simulink model "NavigationSystem"  (R2018b)
settings: Solver=ode4  StartTime=0.0  StopTime=2000  FixedStep=S_time  RelTol=1e-3
InitFcn:
  | run('DataInitial.m')
StopFcn:
  | run('PNPlot.m')
values from neighbouring files (symbols this model uses):
  GM = 3.986e5    (= 398600)    [DataInitial.m]
  N_PN = 5    [DataInitial.m]
  P0_M = [4510.1;4510.1]    [DataInitial.m]
  P0_T = [0;6378.2]    [DataInitial.m]
  V0_M = [2.0056;5.9535]    [DataInitial.m]
  V0_T = [6.7856;2.8801]    [DataInitial.m]
libraries: simulink x1
settings Model: Creator=Administrator  LastModifiedBy=Administrator

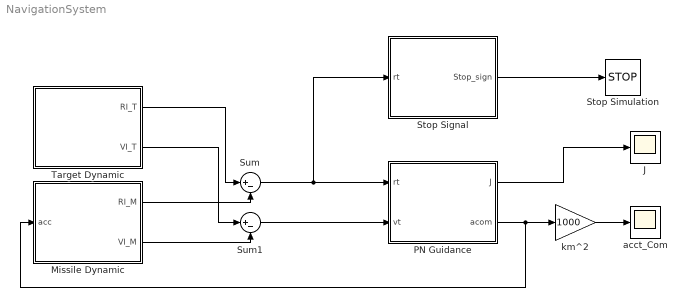
== system NavigationSystem ==
  J : Scope
  Missile Dynamic : Subsystem  mask(导弹设置){P0_M=P0_M, V0_M=V0_M}
      mask prompts: P0_M "导弹初始位置（km）"; V0_M "导弹初始速度（km/s)"
      mask help: 在这里设置导弹的初始位置和速度
  PN Guidance : Subsystem
  Stop Signal : Subsystem
  Stop Simulation : Stop
  Sum : Sum  Inputs=|+-
  Sum1 : Sum  Inputs=|+-
  Target Dynamic : Subsystem  mask(目标设置){P0_T=P0_T, V0_T=V0_T}
      mask prompts: P0_T "目标初始位置（km)"; V0_T "目标初始速度（km/s）"
      mask help: 在这里设置目标的初始位置和速度
  acct_Com : Scope
  km^2 : Gain  Gain=1000
  wires:
  Stop Signal/1(Stop_sign) -> Stop Simulation/1
  Target Dynamic/1(RI_T) -> Sum/1
  Target Dynamic/2(VI_T) -> Sum1/1
  Sum/1 -> Stop Signal/1(rt), PN Guidance/1(rt)
  Sum1/1 -> PN Guidance/2(vt)
  PN Guidance/1(J) -> J/1
  PN Guidance/2(acom) -> Missile Dynamic/1(acc), km^2/1
  km^2/1 -> acct_Com/1
  Missile Dynamic/1(RI_M) -> Sum/2
  Missile Dynamic/2(VI_M) -> Sum1/2

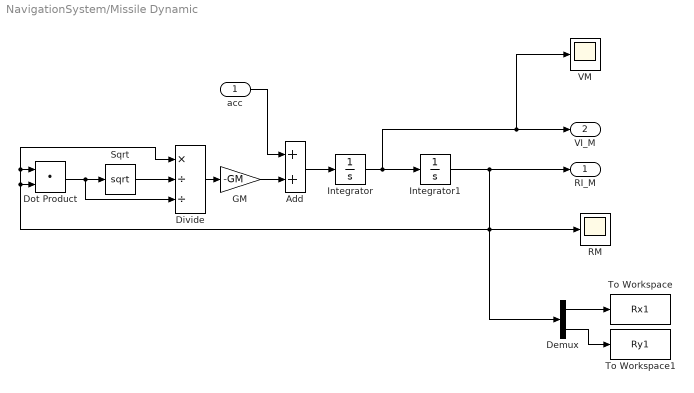
== system NavigationSystem/Missile Dynamic ==
  acc : Inport
  Add : Sum
  Demux : Demux  Outputs=2
  Divide : Product  Inputs=*//
  Dot Product : DotProduct  InputSameDT=on  OutDataTypeStr=Inherit: Inherit via internal rule
  GM : Gain  Gain=-GM
  Integrator : Integrator  InitialCondition=V0_M
  Integrator1 : Integrator  InitialCondition=P0_M
  RM : Scope
  Sqrt : Sqrt  SaturateOnIntegerOverflow=on
  To Workspace : ToWorkspace  VariableName=Rx1  SaveFormat=Timeseries  SampleTime=-1
  To Workspace1 : ToWorkspace  VariableName=Ry1  SaveFormat=Timeseries  SampleTime=-1
  VM : Scope
  RI_M : Outport
  VI_M : Outport  Port=2
  wires:
  Sqrt/1 -> Divide/2
  Integrator/1 -> VM/1, VI_M/1, Integrator1/1
  Dot Product/1 -> Divide/3, Sqrt/1
  Integrator1/1 -> Demux/1, Dot Product/1, Divide/1, Dot Product/2, RM/1, RI_M/1
  Divide/1 -> GM/1
  GM/1 -> Add/2
  Add/1 -> Integrator/1
  acc/1 -> Add/1
  Demux/1 -> To Workspace/1
  Demux/2 -> To Workspace1/1

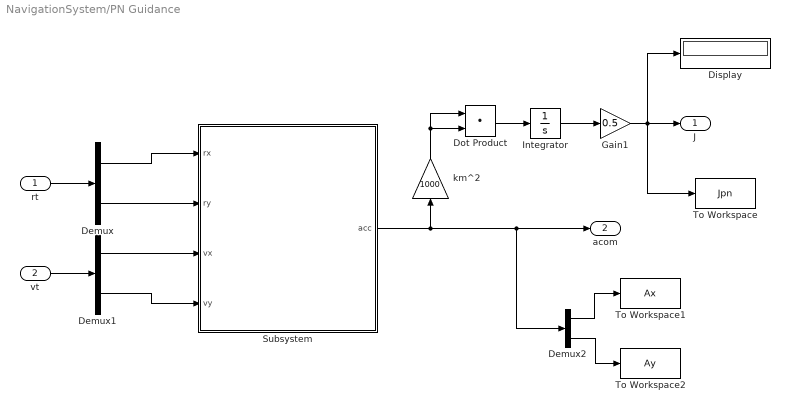
== system NavigationSystem/PN Guidance ==
  rt : Inport
  vt : Inport  Port=2
  Demux : Demux  Outputs=2
  Demux1 : Demux  Outputs=2
  Demux2 : Demux  Outputs=2
  Display : Display
  Dot Product : DotProduct  InputSameDT=on  OutDataTypeStr=Inherit: Inherit via internal rule
  Gain1 : Gain  Gain=0.5
  Integrator : Integrator
  Subsystem : Subsystem
  To Workspace : ToWorkspace  VariableName=Jpn  SaveFormat=Timeseries  SampleTime=-1
  To Workspace1 : ToWorkspace  VariableName=Ax  SaveFormat=Timeseries  SampleTime=-1
  To Workspace2 : ToWorkspace  VariableName=Ay  SaveFormat=Timeseries  SampleTime=-1
  km^2 : Gain  Gain=1000
  J : Outport
  acom : Outport  Port=2
  wires:
  rt/1 -> Demux/1
  Demux/1 -> Subsystem/1(rx)
  Demux/2 -> Subsystem/2(ry)
  vt/1 -> Demux1/1
  Demux1/1 -> Subsystem/3(vx)
  Demux1/2 -> Subsystem/4(vy)
  Dot Product/1 -> Integrator/1
  km^2/1 -> Dot Product/2, Dot Product/1
  Integrator/1 -> Gain1/1
  Gain1/1 -> Display/1, J/1, To Workspace/1
  Demux2/1 -> To Workspace1/1
  Demux2/2 -> To Workspace2/1
  Subsystem/1(acc) -> Demux2/1, acom/1, km^2/1

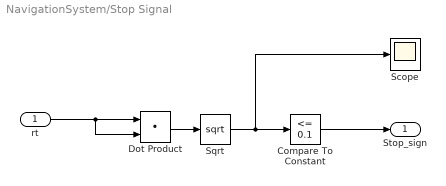
== system NavigationSystem/Stop Signal ==
  rt : Inport
  Compare To Constant : simulink/Logic and Bit Operations/Compare To Constant  relop=<=  const=0.1  OutDataTypeStr=boolean
  Dot Product : DotProduct  InputSameDT=on  OutDataTypeStr=Inherit: Inherit via internal rule
  Scope : Scope
  Sqrt : Sqrt  SaturateOnIntegerOverflow=on
  Stop_sign : Outport
  wires:
  Dot Product/1 -> Sqrt/1
  rt/1 -> Dot Product/1, Dot Product/2
  Sqrt/1 -> Scope/1, Compare To Constant/1
  Compare To Constant/1 -> Stop_sign/1

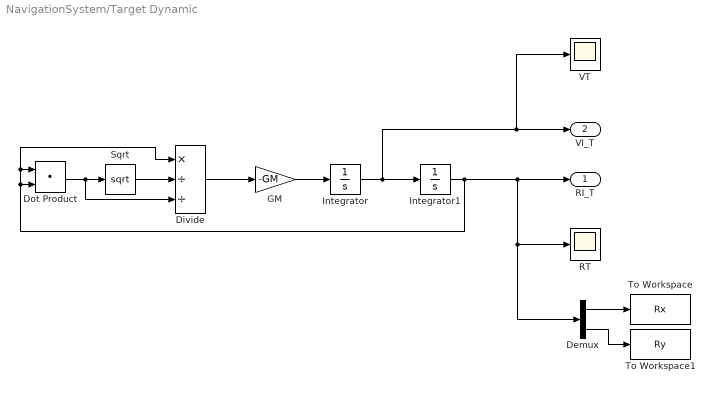
== system NavigationSystem/Target Dynamic ==
  Demux : Demux  Outputs=2
  Divide : Product  Inputs=*//
  Dot Product : DotProduct  InputSameDT=on  OutDataTypeStr=Inherit: Inherit via internal rule
  GM : Gain  Gain=-GM
  Integrator : Integrator  InitialCondition=V0_T
  Integrator1 : Integrator  InitialCondition=P0_T
  RT : Scope
  Sqrt : Sqrt  SaturateOnIntegerOverflow=on
  To Workspace : ToWorkspace  VariableName=Rx  SaveFormat=Timeseries  SampleTime=-1
  To Workspace1 : ToWorkspace  VariableName=Ry  SaveFormat=Timeseries  SampleTime=-1
  VT : Scope
  RI_T : Outport
  VI_T : Outport  Port=2
  wires:
  Integrator/1 -> VT/1, VI_T/1, Integrator1/1
  Integrator1/1 -> Demux/1, RT/1, RI_T/1, Dot Product/1, Divide/1, Dot Product/2
  GM/1 -> Integrator/1
  Divide/1 -> GM/1
  Sqrt/1 -> Divide/2
  Dot Product/1 -> Divide/3, Sqrt/1
  Demux/1 -> To Workspace/1
  Demux/2 -> To Workspace1/1

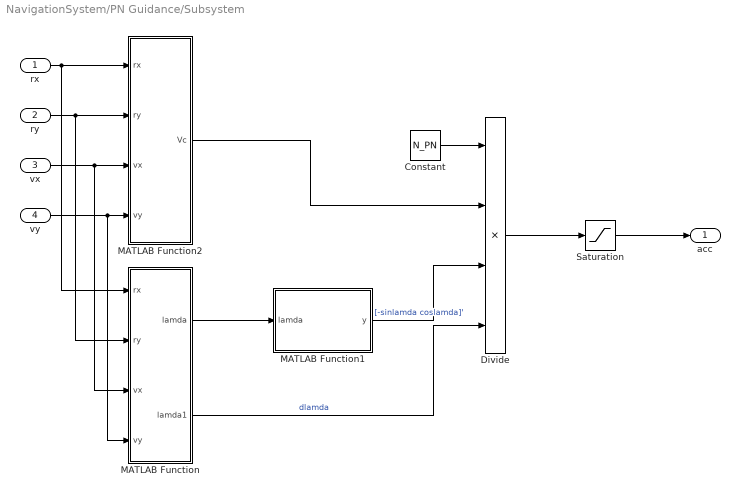
== system NavigationSystem/PN Guidance/Subsystem ==
  rx : Inport
  ry : Inport  Port=2
  vx : Inport  Port=3
  vy : Inport  Port=4
  Constant : Constant  Value=N_PN
  Divide : Product  Inputs=****
  MATLAB Function : MATLAB Function  TreatAsAtomicUnit=on
  MATLAB Function1 : MATLAB Function  TreatAsAtomicUnit=on
  MATLAB Function2 : MATLAB Function  TreatAsAtomicUnit=on
  Saturation : Saturate  UpperLimit=[0.004 0.004]  LowerLimit=[-0.004 -0.004]
  acc : Outport
  wires:
  MATLAB Function/1(lamda) -> MATLAB Function1/1(lamda)
  rx/1 -> MATLAB Function2/1(rx), MATLAB Function/1(rx)
  ry/1 -> MATLAB Function2/2(ry), MATLAB Function/2(ry)
  vx/1 -> MATLAB Function/3(vx), MATLAB Function2/3(vx)
  vy/1 -> MATLAB Function/4(vy), MATLAB Function2/4(vy)
  Divide/1 -> Saturation/1
  MATLAB Function2/1(Vc) -> Divide/2
  Constant/1 -> Divide/1
  MATLAB Function/2(lamda1) -> Divide/4  "dlamda"
  MATLAB Function1/1(y) -> Divide/3  "[-sinlamda coslamda]'"
  Saturation/1 -> acc/1

== matlab function NavigationSystem/PN Guidance/Subsystem/MATLAB Function1 ==
  data: lamda input; y output
function y = sincos(lamda)
y = [-sin(lamda) cos(lamda)]';
end

== matlab function NavigationSystem/PN Guidance/Subsystem/MATLAB Function ==
  data: rx input; lamda output; ry input; vx input; vy input; lamda1 output
function [lamda,lamda1] = LOS(rx,ry,vx,vy)
lamda = atan(ry/rx);
lamda1 = (vy * rx - vx * ry)/(rx^2 + ry^2);
end

== matlab function NavigationSystem/PN Guidance/Subsystem/MATLAB Function2 ==
  data: rx input; Vc output; ry input; vx input; vy input
function Vc = vc(rx,ry,vx,vy)
r=(rx^2+ry^2)^0.5;
Vc=(rx*vx + ry*vy)/r;
end
